simulink model "SimulationKF"  (R2019a)
settings: Solver=VariableStepAuto  StartTime=0.0  StopTime=tmax  RelTol=1e-3
values from neighbouring files (symbols this model uses):
  i = i+1    (= 2)    [PowerRegen.m]    (also in RunSimulation.m = 0; RunSimulationKF.m = -0.005)
  Ki = 20    [RunSimulationKF.m]
  Kp = 600    [RunSimulationKF.m]
  mL = 650    [PowerRegen.m]    (also in RunSimulation.m; RunSimulationKF.m)
  mWz = 1200    [RunSimulation.m]    (also in RunSimulationKF.m)
  P1 = 1e-1    (= 0.1)    [RunSimulationKF.m]
  P2 = (eye(n2) - K2*x2')*P2    [KFLoco.m]    (also in RunSimulationKF.m = 0)
  Pres = 1/1000*[5.7/771 0 1.6]    [RunSimulation.m]    (also in RunSimulationKF.m)
  s0 = 0    [RunSimulation.m]    (also in RunSimulationKF.m)
  smax = 20    [RunSimulationKF.m]
  Ts = 0.01    [RunSimulation.m]    (also in RunSimulationKF.m)
  v0 = 10/3.6    (= 2.77777777778)    [RunSimulation.m]    (also in RunSimulationKF.m)
libraries: simulink x4
settings Model: Creator=raphael  LastModifiedBy=raphael
settings DataIOCC: ReturnWorkspaceOutputs=off
settings DebuggingCC: ArithmeticOperatorsInVariantConditions=warning

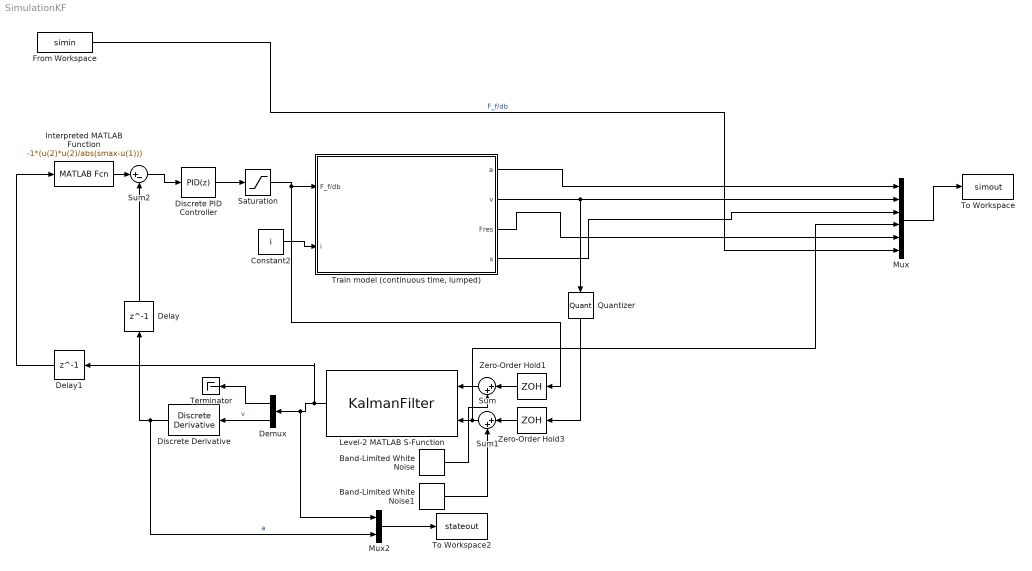
== system SimulationKF ==
  Band-Limited White Noise : simulink/Sources/Band-Limited White Noise  Cov=[P1]  Ts=10*Ts  seed=[43]
  Band-Limited White Noise1 : simulink/Sources/Band-Limited White Noise  Cov=[P2]  Ts=10*Ts  seed=[42]
  Constant2 : Constant  Value=i
  Delay : Delay  DelayLength=1
  Delay1 : Delay  DelayLength=1
  Demux : Demux  Outputs=2
  Discrete Derivative : simulink/Discrete/Discrete Derivative  gainval=-1  ICPrevScaledInput=0.0  OutMin=[]  OutMax=[]  OutDataType=fixdt(1, 16)  OutScaling=2^-10  DoSatur=off
  Discrete PID Controller : simulink/Continuous/PID Controller  Controller=PID  Form=Parallel  TimeDomain=Discrete-time  SampleTime=-1  IntegratorMethod=Forward Euler  FilterMethod=Forward Euler  ControllerParametersSource=internal  P=Kp  I=Ki  D=0  UseFilter=on  N=100  TunerSelectOption=Transfer Function Based (PID Tuner App)  InitialConditionSource=internal  InitialConditionForIntegrator=0  InitialConditionForFilter=0  DifferentiatorICPrevScaledInput=0  ExternalReset=none  TrackingMode=off  Kt=1  LimitOutput=off  UpperSaturationLimit=inf  LowerSaturationLimit=-inf  LinearizeAsGain=off  AntiWindupMode=none  Kb=1  POutMin=[]  POutMax=[]  IOutMin=[]  IOutMax=[]  DOutMin=[]  DOutMax=[]  NOutMin=[]  NOutMax=[]  SumOutMin=[]  SumOutMax=[]  SaturationOutMin=[]  SaturationOutMax=[]  PParamMin=[]  PParamMax=[]  IParamMin=[]  IParamMax=[]  DParamMin=[]  DParamMax=[]  NParamMin=[]  NParamMax=[]  KbParamMin=[]  KbParamMax=[]  KtParamMin=[]  KtParamMax=[]  KbOutMin=[]  KbOutMax=[]  KtOutMin=[]  KtOutMax=[]  IntegratorOutMin=[]  IntegratorOutMax=[]  FilterOutMin=[]  FilterOutMax=[]  SumI1OutMin=[]  SumI1OutMax=[]  SumI2OutMin=[]  SumI2OutMax=[]  SumI3OutMin=[]  SumI3OutMax=[]  SumI4OutMin=[]  SumI4OutMax=[]  SumDOutMin=[]  SumDOutMax=[]  DifferentiatorOutMin=[]  DifferentiatorOutMax=[]  FilterDiffOutCoefMin=[]  FilterDiffOutCoefMax=[]  ReciprocalOutMin=[]  ReciprocalOutMax=[]  SumDenOutMin=[]  SumDenOutMax=[]  SumNumOutMin=[]  SumNumOutMax=[]  DivideOutMin=[]  DivideOutMax=[]  IntegratorContinuousStateAttributes=''  IntegratorStateMustResolveToSignalObject=off  IntegratorRTWStateStorageClass=Auto  FilterContinuousStateAttributes=''  FilterStateMustResolveToSignalObject=off  FilterRTWStateStorageClass=Auto  ParallelPVariant=InternalParameters  IdealPVariant=Disabled  IVariant=InternalParameters  DVariant=InternalParameters  IntegratorVariant=Discrete  SatVariant=Disabled  AWVariant=Passthrough  PCopyVariant=Disabled  TRVariant=Disabled  FdbkBlocksVariant=Forward  IdealPFdbkVariant=Disabled  SatFdbkVariant=Disabled  DerivativeFilterVariant=ForwardEulerFilter  NVariant=InternalParameters  NCopyVariant=Disabled  FilterICVariant=InternalICsFilter  IntegratorICVariant=InternalICs  ExternalResetVariant=Disabled  TRSumVariant=Passthrough  SumFdbkVariant=Disabled  SumVariant=Sum_PID
  From Workspace : FromWorkspace  VariableName=simin  SampleTime=0
  Interpreted MATLAB Function : MATLABFcn  MATLABFcn=-1*(u(2)*u(2)/abs(smax-u(1)))
  Level-2 MATLAB S-Function : M-S-Function  FunctionName=KalmanFilter  Parameters=sysSS.A, sysSS.B, sysSS.C, P, rv, Rw, v0
  Mux : Mux  Inputs=6
  Mux2 : Mux  Inputs=2
  Quantizer : Quantizer  QuantizationInterval=0.8/3.6
  Saturation : Saturate  UpperLimit=0  LowerLimit=-5000
  Sum : Sum  Inputs=|++
  Sum1 : Sum  Inputs=|++
  Sum2 : Sum  Inputs=|+-
  Terminator : Terminator
  To Workspace : ToWorkspace  VariableName=simout  SaveFormat=Timeseries  SampleTime=-1
  To Workspace2 : ToWorkspace  VariableName=stateout  SaveFormat=Timeseries  SampleTime=-1
  "Train model (continuous time, lumped)" : Subsystem
  Zero-Order Hold1 : ZeroOrderHold  SampleTime=Ts
  Zero-Order Hold3 : ZeroOrderHold  SampleTime=Ts
  wires:
  From Workspace/1 -> Mux/6  "F_f/db"
  Mux/1 -> To Workspace/1
  "Train model (continuous time, lumped)"/4(s) -> Mux/3
  "Train model (continuous time, lumped)"/3(Fres) -> Mux/5
  Constant2/1 -> "Train model (continuous time, lumped)"/2(i)
  "Train model (continuous time, lumped)"/1(a) -> Mux/1
  Level-2 MATLAB S-Function/1 -> Delay1/1, Mux2/1, Demux/1
  Demux/2 -> Discrete Derivative/1  "v"
  Discrete Derivative/1 -> Mux2/2, Delay/1  "a"
  Discrete PID Controller/1 -> Saturation/1
  Mux2/1 -> To Workspace2/1
  Delay/1 -> Sum2/2
  Saturation/1 -> Zero-Order Hold1/1, "Train model (continuous time, lumped)"/1(F_f/db)
  Interpreted MATLAB Function/1 -> Sum2/1
  Delay1/1 -> Interpreted MATLAB Function/1
  Demux/1 -> Terminator/1
  Zero-Order Hold1/1 -> Sum/1
  Sum/1 -> Level-2 MATLAB S-Function/1
  Sum1/1 -> Mux/4, Level-2 MATLAB S-Function/2
  Zero-Order Hold3/1 -> Sum1/1
  Band-Limited White Noise/1 -> Sum/2
  Band-Limited White Noise1/1 -> Sum1/2
  Sum2/1 -> Discrete PID Controller/1
  "Train model (continuous time, lumped)"/2(v) -> Mux/2, Quantizer/1
  Quantizer/1 -> Zero-Order Hold3/1

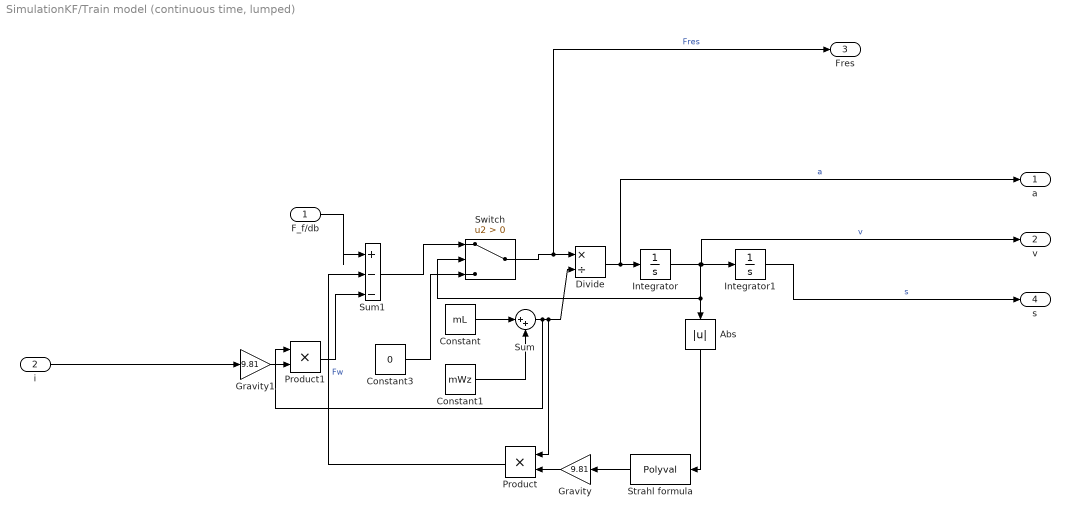
== system SimulationKF/Train model (continuous time, lumped) ==
  F_f/db : Inport
  i : Inport  Port=2
  Abs : Abs
  Constant : Constant  Value=mL
  Constant1 : Constant  Value=mWz
  Constant3 : Constant  Value=0
  Divide : Product  Inputs=*/
  Gravity : Gain  Gain=9.81
  Gravity1 : Gain  Gain=9.81
  Integrator : Integrator  InitialCondition=v0
  Integrator1 : Integrator  InitialCondition=s0
  Product : Product
  Product1 : Product
  Strahl formula : Polyval  Coefs=Pres
  Sum : Sum  Inputs=|++
  Sum1 : Sum  Inputs=|+--
  Switch : Switch  Criteria=u2 > Threshold
  a : Outport
  v : Outport  Port=2
  Fres : Outport  Port=3
  s : Outport  Port=4
  wires:
  Switch/1 -> Fres/1, Divide/1  "Fres"
  Integrator1/1 -> s/1  "s"
  Constant3/1 -> Switch/3
  Product1/1 -> Sum1/3
  Constant1/1 -> Sum/2
  Strahl formula/1 -> Gravity/1
  Abs/1 -> Strahl formula/1
  Gravity1/1 -> Product1/2
  F_f/db/1 -> Sum1/1
  Gravity/1 -> Product/2
  Product/1 -> Sum1/2  "Fw"
  Constant/1 -> Sum/1
  Integrator/1 -> v/1, Integrator1/1, Switch/2, Abs/1  "v"
  Sum/1 -> Product1/1, Product/1, Divide/2
  Divide/1 -> a/1, Integrator/1  "a"
  Sum1/1 -> Switch/1
  i/1 -> Gravity1/1
